simulink model "LdAfsDblSlave"  (R2020b)
settings: configuration reference "VLS_Standard_Configuration" (kept outside this file)
undefined symbols (not defined in the file): C_AfsRampTimeMatrix, C_CieCurveGammaToPwmY, C_CieCurvePwmToGammaY, C_DblLeftAngles, C_DblRampTime, C_DblRightAngles, C_DblSlavePeriod, C_EndIndexOfEachLightingModule, C_IsDblActive, C_LedCenterDist, C_LedCenterLimits, C_LedLeftDist, C_LedRightDist, C_StartIndexOfEachLightingModule
libraries: AfsSlaveLib x1, DblSlaveLib x1
settings Model: DataDictionary=LdAfsDblSlaveDD.sldd  Creator=ahashem  LastModifiedBy=ahashem
settings ConfigSetRef: SourceName=VLS_Standard_Configuration

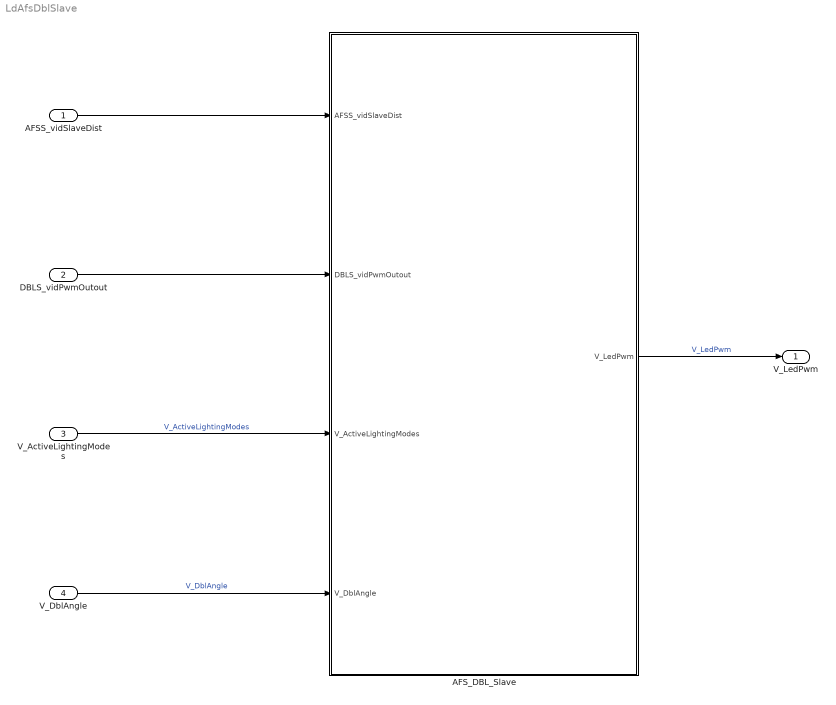
== system LdAfsDblSlave ==
  AFSS_vidSlaveDist : Inport  OutputFunctionCall=on
  DBLS_vidPwmOutout : Inport  Port=2  OutputFunctionCall=on
  V_ActiveLightingModes : Inport  Port=3
  V_DblAngle : Inport  Port=4
  AFS_DBL_Slave : Subsystem  Description=ADB_Master subsystem
  V_LedPwm : Outport  VectorParamsAs1DForOutWhenUnconnected=off
  wires:
  AFSS_vidSlaveDist/1 -> AFS_DBL_Slave/1(AFSS_vidSlaveDist)
  DBLS_vidPwmOutout/1 -> AFS_DBL_Slave/2(DBLS_vidPwmOutout)
  V_ActiveLightingModes/1 -> AFS_DBL_Slave/3(V_ActiveLightingModes)  "V_ActiveLightingModes"
  V_DblAngle/1 -> AFS_DBL_Slave/4(V_DblAngle)  "V_DblAngle"
  AFS_DBL_Slave/1(V_LedPwm) -> V_LedPwm/1  "V_LedPwm"

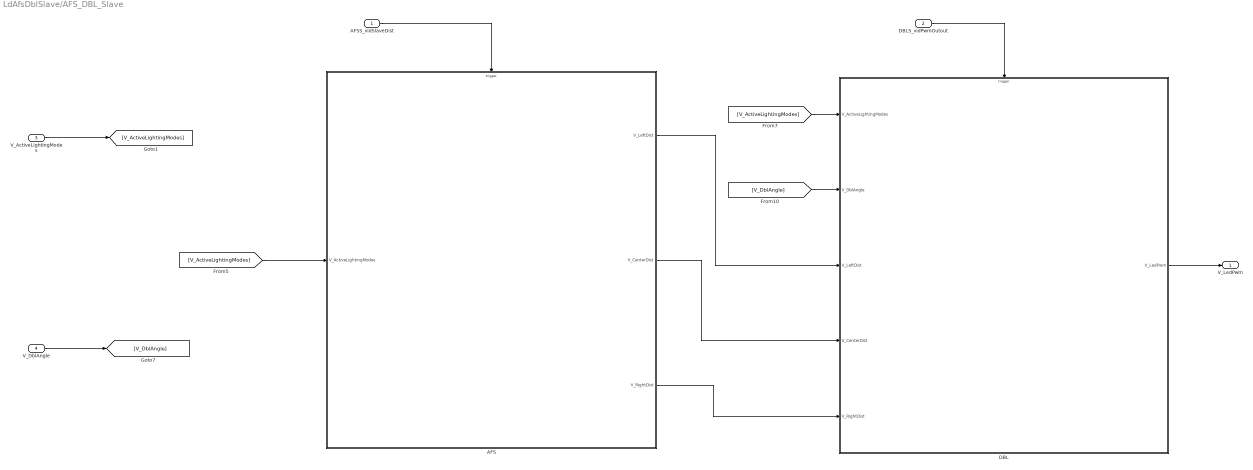
== system LdAfsDblSlave/AFS_DBL_Slave ==
  AFSS_vidSlaveDist : Inport
  DBLS_vidPwmOutout : Inport  Port=2
  V_ActiveLightingModes : Inport  Port=3
  V_DblAngle : Inport  Port=4
  AFS : Subsystem  Description=Clustering subsystem
  DBL : Subsystem  Description=Clustering subsystem
  V_LedPwm : Outport  VectorParamsAs1DForOutWhenUnconnected=off
  wires:
  AFSS_vidSlaveDist/1 -> AFS/Trigger
  DBLS_vidPwmOutout/1 -> DBL/Trigger
  V_ActiveLightingModes/1 -> [V_ActiveLightingModes]
  AFS/2(V_CenterDist) -> DBL/4(V_CenterDist)
  AFS/1(V_LeftDist) -> DBL/3(V_LeftDist)
  AFS/3(V_RightDist) -> DBL/5(V_RightDist)
  [V_ActiveLightingModes] -> AFS/1(V_ActiveLightingModes)
  [V_ActiveLightingModes] -> DBL/1(V_ActiveLightingModes)
  V_DblAngle/1 -> [V_DblAngle]
  [V_DblAngle] -> DBL/2(V_DblAngle)
  DBL/1(V_LedPwm) -> V_LedPwm/1

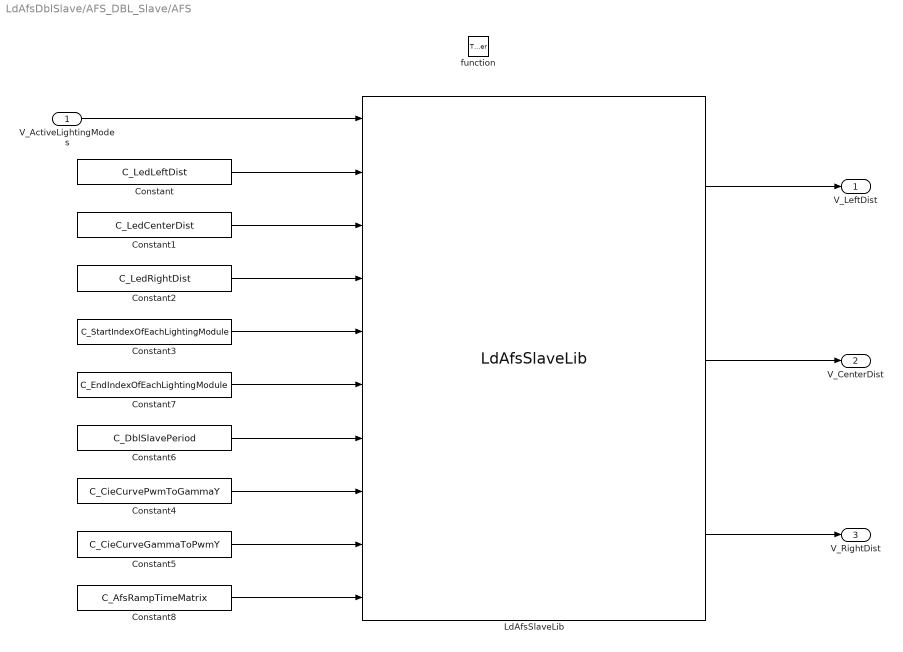
== system LdAfsDblSlave/AFS_DBL_Slave/AFS ==
  V_ActiveLightingModes : Inport
  function : TriggerPort  TriggerType=function-call  VariantControl=Variant
      settings: AttributesFormatString=StatesWhenEnabling: %<StatesWhenEnabling>
  Constant : Constant  Value=C_LedLeftDist
  Constant1 : Constant  Value=C_LedCenterDist
  Constant2 : Constant  Value=C_LedRightDist
  Constant3 : Constant  Value=C_StartIndexOfEachLightingModule
  Constant4 : Constant  Value=C_CieCurvePwmToGammaY
  Constant5 : Constant  Value=C_CieCurveGammaToPwmY
  Constant6 : Constant  Value=C_DblSlavePeriod
  Constant7 : Constant  Value=C_EndIndexOfEachLightingModule
  Constant8 : Constant  Value=C_AfsRampTimeMatrix
  LdAfsSlaveLib : AfsSlaveLib/LdAfsSlaveLib  SystemSampleTime=-1  VariantActivationTime=update diagram  Latency=0  AutoFrameSizeCalculation=off
  V_LeftDist : Outport  VectorParamsAs1DForOutWhenUnconnected=off
  V_CenterDist : Outport  Port=2  VectorParamsAs1DForOutWhenUnconnected=off
  V_RightDist : Outport  Port=3  VectorParamsAs1DForOutWhenUnconnected=off
  wires:
  V_ActiveLightingModes/1 -> LdAfsSlaveLib/1
  LdAfsSlaveLib/3 -> V_RightDist/1
  LdAfsSlaveLib/2 -> V_CenterDist/1
  LdAfsSlaveLib/1 -> V_LeftDist/1
  Constant/1 -> LdAfsSlaveLib/2
  Constant1/1 -> LdAfsSlaveLib/3
  Constant2/1 -> LdAfsSlaveLib/4
  Constant3/1 -> LdAfsSlaveLib/5
  Constant7/1 -> LdAfsSlaveLib/6
  Constant6/1 -> LdAfsSlaveLib/7
  Constant4/1 -> LdAfsSlaveLib/8
  Constant5/1 -> LdAfsSlaveLib/9
  Constant8/1 -> LdAfsSlaveLib/10

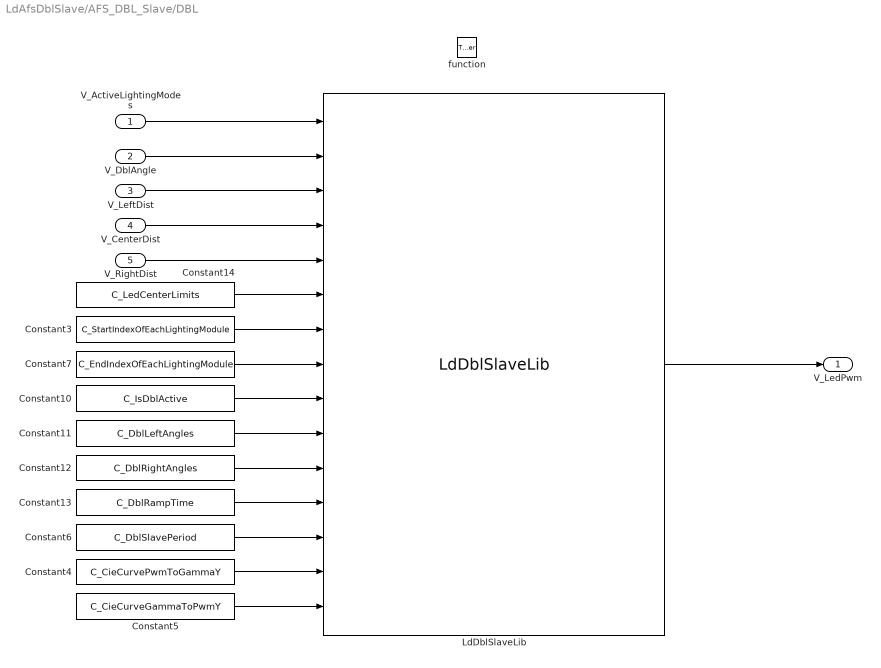
== system LdAfsDblSlave/AFS_DBL_Slave/DBL ==
  V_ActiveLightingModes : Inport
  V_DblAngle : Inport  Port=2
  V_LeftDist : Inport  Port=3
  V_CenterDist : Inport  Port=4
  V_RightDist : Inport  Port=5
  function : TriggerPort  TriggerType=function-call  VariantControl=Variant
      settings: AttributesFormatString=StatesWhenEnabling: %<StatesWhenEnabling>
  Constant10 : Constant  Value=C_IsDblActive
  Constant11 : Constant  Value=C_DblLeftAngles
  Constant12 : Constant  Value=C_DblRightAngles
  Constant13 : Constant  Value=C_DblRampTime
  Constant14 : Constant  Value=C_LedCenterLimits
  Constant3 : Constant  Value=C_StartIndexOfEachLightingModule
  Constant4 : Constant  Value=C_CieCurvePwmToGammaY
  Constant5 : Constant  Value=C_CieCurveGammaToPwmY
  Constant6 : Constant  Value=C_DblSlavePeriod
  Constant7 : Constant  Value=C_EndIndexOfEachLightingModule
  LdDblSlaveLib : DblSlaveLib/LdDblSlaveLib  SystemSampleTime=-1  VariantActivationTime=update diagram  Latency=0  AutoFrameSizeCalculation=off
      link override DblCalc/ActiveModule/DblActive/MultiLed/Selector: IndexMode=One-based
  V_LedPwm : Outport  VectorParamsAs1DForOutWhenUnconnected=off
  wires:
  V_ActiveLightingModes/1 -> LdDblSlaveLib/1
  V_DblAngle/1 -> LdDblSlaveLib/2
  V_CenterDist/1 -> LdDblSlaveLib/4
  V_RightDist/1 -> LdDblSlaveLib/5
  V_LeftDist/1 -> LdDblSlaveLib/3
  LdDblSlaveLib/1 -> V_LedPwm/1
  Constant6/1 -> LdDblSlaveLib/13
  Constant4/1 -> LdDblSlaveLib/14
  Constant13/1 -> LdDblSlaveLib/12
  Constant5/1 -> LdDblSlaveLib/15
  Constant12/1 -> LdDblSlaveLib/11
  Constant11/1 -> LdDblSlaveLib/10
  Constant10/1 -> LdDblSlaveLib/9
  Constant7/1 -> LdDblSlaveLib/8
  Constant3/1 -> LdDblSlaveLib/7
  Constant14/1 -> LdDblSlaveLib/6
